simulink model "BG"  (R2014a)
settings: Solver=ode3  StartTime=0.0  StopTime=1  FixedStep=dt  MaxStep=dt  RelTol=1e-3
values from neighbouring files (symbols this model uses):
  a1 = .4    (= 0.4)    [parameters.m]
  a2 = .35    (= 0.35)    [parameters.m]
  a3 = .25    (= 0.25)    [parameters.m]
  aTc = 0.05    [parameters.m]
  dt = 1e-3    (= 0.001)    [parameters.m]
  g = 1    [parameters.m]
  K = 1    [parameters.m]
  mTc = 0.01    [parameters.m]
  OP1_0 = [ax1_0 ay1_0 0]    [parameters.m]
  OP2_0 = OP1_0 + P1P2_0    [parameters.m]
  OP3_0 = OP2_0 + P2P3_0    [parameters.m]
  OT = [xf yf 0]    [animation.m]    (also in parameters.m = [0.5 0.5 0])
  OT_cercle = [0.6 0.55 0]    [parameters.m]
  p1 = w2 + w3    (= 3)    [parameters.m]
  P1P2_0 = [ax2_0 ay2_0 0]    [parameters.m]
  p2 = w1 + w3    (= 4)    [parameters.m]
  P2P3_0 = [ax3_0 ay3_0 0]    [parameters.m]
  p3 = w2 + w1    (= 5)    [parameters.m]
  tau = 0.001    [parameters.m]
  theta1_0 = zero_vector    [parameters.m]
  theta2_0 = zero_vector    [parameters.m]
  theta3_0 = zero_vector    [parameters.m]
  Vmax = 30    [parameters.m]
  w1 = 3    [parameters.m]
  w2 = 2    [parameters.m]
  w3 = 1    [parameters.m]
  zero_vector = [0 0 0]    [parameters.m]
libraries: vrlib x9, simulink x1
(part 3 of 4)

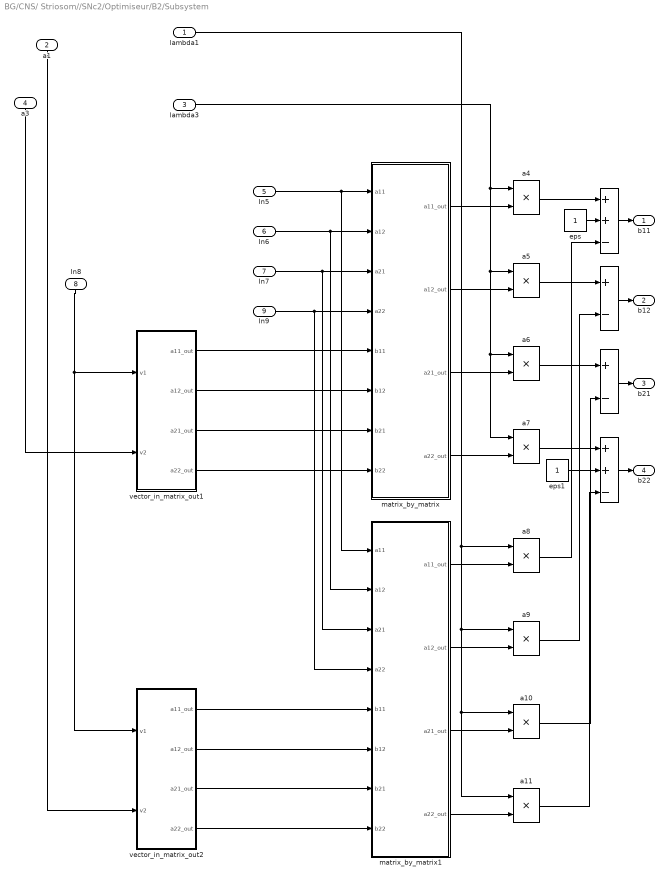
== system BG/CNS/ Striosom//SNc2/Optimiseur/B2/Subsystem ==
  lambda1 : Inport
  a1 : Inport  Port=2
  lambda3 : Inport  Port=3
  a3 : Inport  Port=4
  In5 : Inport  Port=5
  In6 : Inport  Port=6
  In7 : Inport  Port=7
  In8 : Inport  Port=8
  In9 : Inport  Port=9
  "                                                                                                    " : Sum  Inputs=++-
  "                                                                                                      " : Sum  Inputs=++-
  "                                                                                                       " : Sum  Inputs=+-
  "                                                                                                           " : Sum  Inputs=+-
  a{4..11} (8 alike) : Product
  eps : Constant
  eps1 : Constant
  matrix_by_matrix : Subsystem
  matrix_by_matrix1 : Subsystem
  vector_in_matrix_out1 : Subsystem
  vector_in_matrix_out2 : Subsystem
  b11 : Outport
  b12 : Outport  Port=2
  b21 : Outport  Port=3
  b22 : Outport  Port=4
  wires:
  In5/1 -> matrix_by_matrix1/1(a11), matrix_by_matrix/1(a11)
  In6/1 -> matrix_by_matrix1/2(a12), matrix_by_matrix/2(a12)
  In7/1 -> matrix_by_matrix1/3(a21), matrix_by_matrix/3(a21)
  In9/1 -> matrix_by_matrix1/4(a22), matrix_by_matrix/4(a22)
  vector_in_matrix_out1/4(a22_out) -> matrix_by_matrix/8(b22)
  vector_in_matrix_out1/3(a21_out) -> matrix_by_matrix/7(b21)
  vector_in_matrix_out1/1(a11_out) -> matrix_by_matrix/5(b11)
  vector_in_matrix_out1/2(a12_out) -> matrix_by_matrix/6(b12)
  matrix_by_matrix/1(a11_out) -> a4/2
  lambda3/1 -> a7/1, a6/1, a5/1, a4/1
  matrix_by_matrix/2(a12_out) -> a5/2
  matrix_by_matrix/3(a21_out) -> a6/2
  matrix_by_matrix/4(a22_out) -> a7/2
  vector_in_matrix_out2/2(a12_out) -> matrix_by_matrix1/6(b12)
  vector_in_matrix_out2/3(a21_out) -> matrix_by_matrix1/7(b21)
  vector_in_matrix_out2/1(a11_out) -> matrix_by_matrix1/5(b11)
  vector_in_matrix_out2/4(a22_out) -> matrix_by_matrix1/8(b22)
  matrix_by_matrix1/1(a11_out) -> a8/2
  matrix_by_matrix1/2(a12_out) -> a9/2
  matrix_by_matrix1/3(a21_out) -> a10/2
  matrix_by_matrix1/4(a22_out) -> a11/2
  lambda1/1 -> a11/1, a10/1, a9/1, a8/1
  a4/1 -> "                                                                                                    "/1
  a8/1 -> "                                                                                                    "/3
  eps/1 -> "                                                                                                    "/2
  a5/1 -> "                                                                                                       "/1
  a9/1 -> "                                                                                                       "/2
  a6/1 -> "                                                                                                           "/1
  a10/1 -> "                                                                                                           "/2
  a7/1 -> "                                                                                                      "/1
  eps1/1 -> "                                                                                                      "/2
  a11/1 -> "                                                                                                      "/3
  a1/1 -> vector_in_matrix_out2/2(v2)
  "                                                                                                       "/1 -> b12/1
  "                                                                                                           "/1 -> b21/1
  a3/1 -> vector_in_matrix_out1/2(v2)
  "                                                                                                      "/1 -> b22/1
  "                                                                                                    "/1 -> b11/1
  In8/1 -> vector_in_matrix_out2/1(v1), vector_in_matrix_out1/1(v1)

== system BG/CNS/ Striosom//SNc2/Optimiseur/B2/inverse_matrix ==
  a11 : Inport
  a12 : Inport  Port=2
  a21 : Inport  Port=3
  a22 : Inport  Port=4
  "                                                                                                    " : Sum  Inputs=+-+
  Divide{1..4} (4 alike) : Product  Inputs=*/
  Gain : Gain  Gain=-1
  Gain1 : Gain  Gain=-1
  a1 : Product
  a2 : Product
  eps : Constant  Value=1e-4
  a11_out : Outport
  a12_out : Outport  Port=2
  a21_out : Outport  Port=3
  a22_out : Outport  Port=4
  wires:
  a11/1 -> Divide2/1, a1/1
  a22/1 -> Divide1/1, a1/2
  a12/1 -> a2/1, Gain1/1
  a21/1 -> Gain/1, a2/2
  a1/1 -> "                                                                                                    "/1
  a2/1 -> "                                                                                                    "/2
  "                                                                                                    "/1 -> Divide1/2, Divide2/2, Divide3/2, Divide4/2
  Divide1/1 -> a11_out/1
  Divide2/1 -> a22_out/1
  Divide3/1 -> a12_out/1
  Divide4/1 -> a21_out/1
  Gain/1 -> Divide4/1
  Gain1/1 -> Divide3/1
  eps/1 -> "                                                                                                    "/3

== system BG/CNS/ Striosom//SNc2/Optimiseur/B2/vector_in_matrix_out ==
  v1 : Inport
  v2 : Inport  Port=2
  Demux : Demux  Outputs=3
  Demux1 : Demux  Outputs=3
  a{11..12,21..22} (4 alike) : Product
  a11_out : Outport
  a12_out : Outport  Port=2
  a21_out : Outport  Port=3
  a22_out : Outport  Port=4
  wires:
  v1/1 -> Demux/1
  v2/1 -> Demux1/1
  a11/1 -> a11_out/1
  Demux/1 -> a12/1, a11/1
  a12/1 -> a12_out/1
  a21/1 -> a21_out/1
  Demux/2 -> a22/1, a21/1
  a22/1 -> a22_out/1
  Demux1/1 -> a11/2, a21/2
  Demux1/2 -> a22/2, a12/2

== system BG/CNS/ Striosom//SNc2/Optimiseur/lambda/alpha ==
  d : Inport
  c1 : Inport  Port=2
  c2 : Inport  Port=3
  c3 : Inport  Port=4
  "                                                                                                    " : Sum
  Divide1 : Product  Inputs=*/
  Divide2 : Product  Inputs=*/
  Divide3 : Product  Inputs=*/
  Gain : Gain  Gain=w2*w3
  Gain1 : Gain  Gain=w1*w3
  Gain2 : Gain  Gain=w2*w1
  eps : Constant  Value=1e-2
  alpha1 : Outport
  alpha2 : Outport  Port=2
  alpha3 : Outport  Port=3
  wires:
  c1/1 -> Divide1/1
  d/1 -> "                                                                                                    "/1
  eps/1 -> "                                                                                                    "/2
  Divide1/1 -> Gain/1
  "                                                                                                    "/1 -> Divide3/2, Divide2/2, Divide1/2
  c2/1 -> Divide2/1
  Divide2/1 -> Gain1/1
  Divide3/1 -> Gain2/1
  c3/1 -> Divide3/1
  Gain/1 -> alpha1/1
  Gain1/1 -> alpha2/1
  Gain2/1 -> alpha3/1

== system BG/CNS/ Striosom//SNc2/Optimiseur/lambda/d=V^T(VV^T)^-1V ==
  In1 : Inport
  Dot Product : DotProduct  InputSameDT=on  OutDataTypeStr=Inherit: Inherit via internal rule
  inverse_matrix : Subsystem
  matrix_vector_multiplication : Subsystem
  vector_in_matrix_out : Subsystem
  d : Outport
  wires:
  vector_in_matrix_out/4(a22_out) -> inverse_matrix/4(a22)
  vector_in_matrix_out/2(a12_out) -> inverse_matrix/2(a12)
  vector_in_matrix_out/1(a11_out) -> inverse_matrix/1(a11)
  matrix_vector_multiplication/1(vec_out) -> Dot Product/2
  vector_in_matrix_out/3(a21_out) -> inverse_matrix/3(a21)
  inverse_matrix/2(a12_out) -> matrix_vector_multiplication/2(a12)
  In1/1 -> Dot Product/1, matrix_vector_multiplication/5(v1), vector_in_matrix_out/2(v2), vector_in_matrix_out/1(v1)
  inverse_matrix/3(a21_out) -> matrix_vector_multiplication/3(a21)
  inverse_matrix/1(a11_out) -> matrix_vector_multiplication/1(a11)
  inverse_matrix/4(a22_out) -> matrix_vector_multiplication/4(a22)
  Dot Product/1 -> d/1

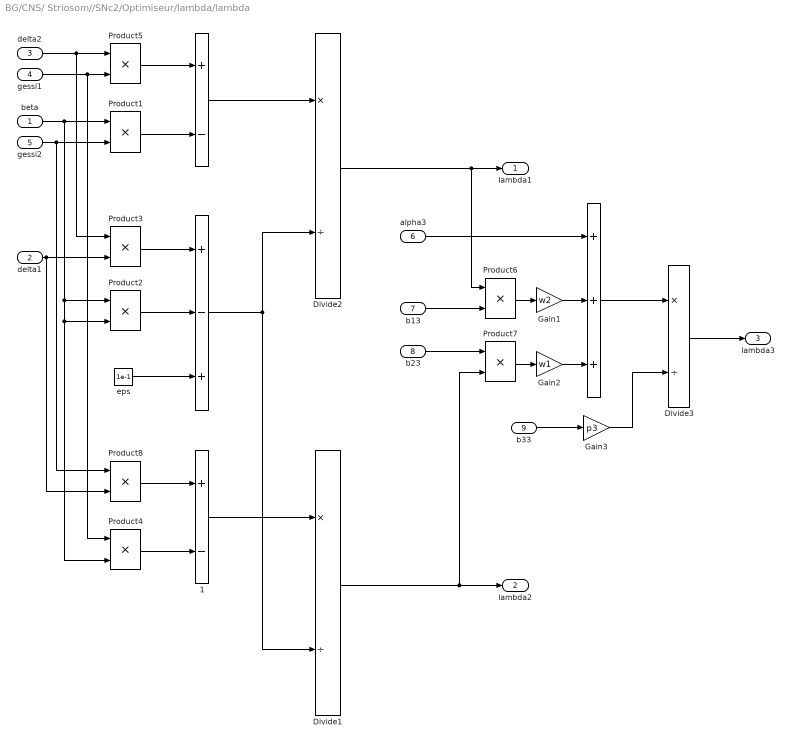
== system BG/CNS/ Striosom//SNc2/Optimiseur/lambda/lambda ==
  beta : Inport
  delta1 : Inport  Port=2
  delta2 : Inport  Port=3
  gessi1 : Inport  Port=4
  gessi2 : Inport  Port=5
  alpha3 : Inport  Port=6
  b13 : Inport  Port=7
  b23 : Inport  Port=8
  b33 : Inport  Port=9
  "                                                                                                        " : Sum  Inputs=+-
  "                                                                                                           " : Sum  Inputs=+-+
  "                                                                                                                 " : Sum  Inputs=+++
  "                                                                                                        1" : Sum  Inputs=+-
  Divide1 : Product  Inputs=*/
  Divide2 : Product  Inputs=*/
  Divide3 : Product  Inputs=*/
  Gain1 : Gain  Gain=w2
  Gain2 : Gain  Gain=w1
  Gain3 : Gain  Gain=p3
  Product{1..8} (8 alike) : Product
  eps : Constant  Value=1e-1
  lambda1 : Outport
  lambda2 : Outport  Port=2
  lambda3 : Outport  Port=3
  wires:
  delta2/1 -> Product3/1, Product5/1
  Product5/1 -> "                                                                                                        "/1
  Product1/1 -> "                                                                                                        "/2
  Product3/1 -> "                                                                                                           "/1
  Product2/1 -> "                                                                                                           "/2
  eps/1 -> "                                                                                                           "/3
  "                                                                                                        "/1 -> Divide2/1
  "                                                                                                           "/1 -> Divide2/2, Divide1/2
  Divide2/1 -> Product6/1, lambda1/1
  gessi2/1 -> Product8/1, Product1/2
  delta1/1 -> Product8/2, Product3/2
  gessi1/1 -> Product4/1, Product5/2
  beta/1 -> Product2/2, Product4/2, Product2/1, Product1/1
  Product8/1 -> "                                                                                                        1"/1
  Product4/1 -> "                                                                                                        1"/2
  "                                                                                                        1"/1 -> Divide1/1
  Divide1/1 -> Product7/2, lambda2/1
  b13/1 -> Product6/2
  b23/1 -> Product7/1
  Product7/1 -> Gain2/1
  Product6/1 -> Gain1/1
  alpha3/1 -> "                                                                                                                 "/1
  "                                                                                                                 "/1 -> Divide3/1
  b33/1 -> Gain3/1
  Gain3/1 -> Divide3/2
  Divide3/1 -> lambda3/1
  Gain1/1 -> "                                                                                                                 "/2
  Gain2/1 -> "                                                                                                                 "/3

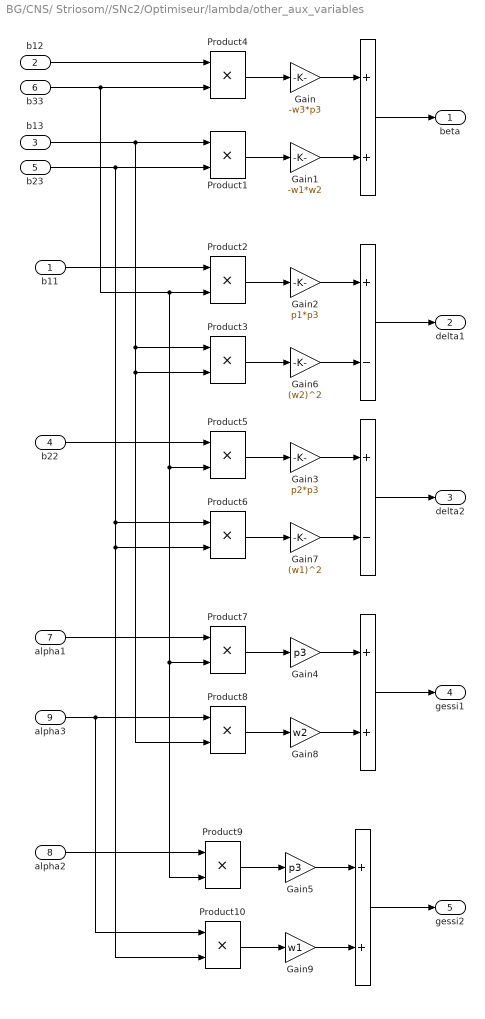
== system BG/CNS/ Striosom//SNc2/Optimiseur/lambda/other_aux_variables ==
  b11 : Inport
  b12 : Inport  Port=2
  b13 : Inport  Port=3
  b22 : Inport  Port=4
  b23 : Inport  Port=5
  b33 : Inport  Port=6
  alpha1 : Inport  Port=7
  alpha2 : Inport  Port=8
  alpha3 : Inport  Port=9
  "                                                                                                    " : Sum
  "                                                                                                     " : Sum  Inputs=+-
  "                                                                                                        " : Sum  Inputs=+-
  "                                                                                                                          " : Sum
  "                                                                                                                               " : Sum
  Gain : Gain  Gain=-w3*p3
  Gain1 : Gain  Gain=-w1*w2
  Gain2 : Gain  Gain=p1*p3
  Gain3 : Gain  Gain=p2*p3
  Gain4 : Gain  Gain=p3
  Gain5 : Gain  Gain=p3
  Gain6 : Gain  Gain=(w2)^2
  Gain7 : Gain  Gain=(w1)^2
  Gain8 : Gain  Gain=w2
  Gain9 : Gain  Gain=w1
  Product{1..10} (10 alike) : Product
  beta : Outport
  delta1 : Outport  Port=2
  delta2 : Outport  Port=3
  gessi1 : Outport  Port=4
  gessi2 : Outport  Port=5
  wires:
  b12/1 -> Product4/1
  Product4/1 -> Gain/1
  Product1/1 -> Gain1/1
  Gain/1 -> "                                                                                                    "/1
  Gain1/1 -> "                                                                                                    "/2
  "                                                                                                    "/1 -> beta/1
  Product2/1 -> Gain2/1
  b11/1 -> Product2/1
  Gain2/1 -> "                                                                                                     "/1
  Product3/1 -> Gain6/1
  "                                                                                                     "/1 -> delta1/1
  b23/1 -> Product6/1, Product10/2, Product6/2, Product1/2
  Product5/1 -> Gain3/1
  b22/1 -> Product5/1
  Gain3/1 -> "                                                                                                        "/1
  Product6/1 -> Gain7/1
  "                                                                                                        "/1 -> delta2/1
  b33/1 -> Product9/2, Product7/2, Product5/2, Product2/2, Product4/2
  alpha3/1 -> Product10/1, Product8/1
  b13/1 -> Product8/2, Product3/2, Product3/1, Product1/1
  Product7/1 -> Gain4/1
  alpha1/1 -> Product7/1
  Gain4/1 -> "                                                                                                                          "/1
  Product8/1 -> Gain8/1
  "                                                                                                                          "/1 -> gessi1/1
  Product9/1 -> Gain5/1
  Gain5/1 -> "                                                                                                                               "/1
  Product10/1 -> Gain9/1
  "                                                                                                                               "/1 -> gessi2/1
  alpha2/1 -> Product9/1
  Gain6/1 -> "                                                                                                     "/2
  Gain7/1 -> "                                                                                                        "/2
  Gain8/1 -> "                                                                                                                          "/2
  Gain9/1 -> "                                                                                                                               "/2

== system BG/CNS/ Striosom//SNc2/Optimiseur/lambda/producing_dot_productions ==
  v : Inport
  a1 : Inport  Port=2
  a2 : Inport  Port=3
  a3 : Inport  Port=4
  Dot Product{,1..8} (9 alike) : DotProduct  InputSameDT=on  OutDataTypeStr=Inherit: Inherit via internal rule
  c1 : Outport
  c2 : Outport  Port=2
  c3 : Outport  Port=3
  b11 : Outport  Port=4
  b12 : Outport  Port=5
  b13 : Outport  Port=6
  b22 : Outport  Port=7
  b23 : Outport  Port=8
  b33 : Outport  Port=9
  wires:
  Dot Product/1 -> c1/1
  v/1 -> Dot Product2/1, Dot Product1/1, Dot Product/1
  a1/1 -> Dot Product4/1, Dot Product5/1, Dot Product3/2, Dot Product3/1, Dot Product/2
  Dot Product1/1 -> c2/1
  a2/1 -> Dot Product7/1, Dot Product6/2, Dot Product6/1, Dot Product4/2, Dot Product1/2
  Dot Product2/1 -> c3/1
  a3/1 -> Dot Product5/2, Dot Product7/2, Dot Product8/1, Dot Product8/2, Dot Product2/2
  Dot Product3/1 -> b11/1
  Dot Product4/1 -> b12/1
  Dot Product5/1 -> b13/1
  Dot Product6/1 -> b22/1
  Dot Product7/1 -> b23/1
  Dot Product8/1 -> b33/1

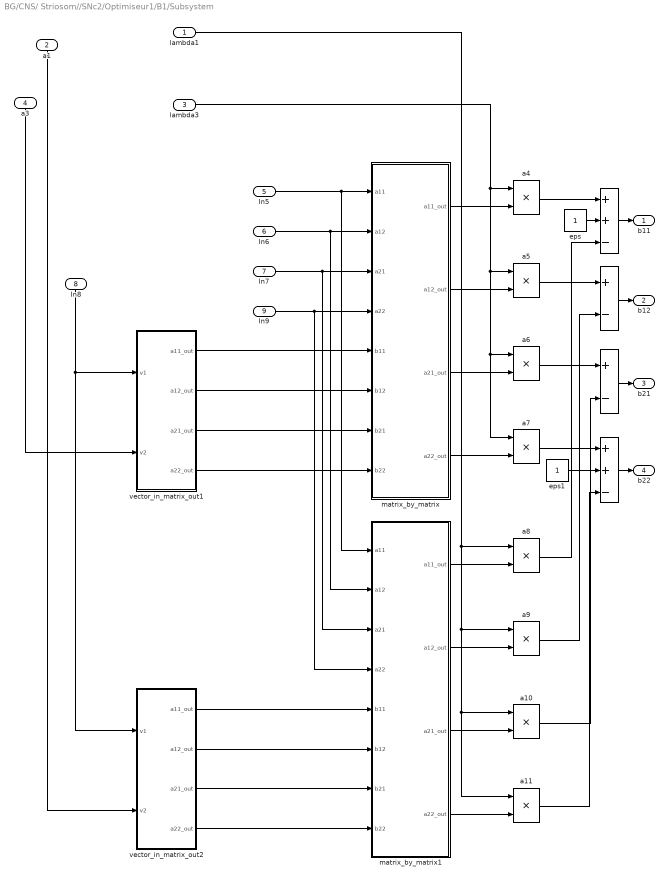
== system BG/CNS/ Striosom//SNc2/Optimiseur1/B1/Subsystem ==
  lambda1 : Inport
  a1 : Inport  Port=2
  lambda3 : Inport  Port=3
  a3 : Inport  Port=4
  In5 : Inport  Port=5
  In6 : Inport  Port=6
  In7 : Inport  Port=7
  In8 : Inport  Port=8
  In9 : Inport  Port=9
  "                                                                                                    " : Sum  Inputs=++-
  "                                                                                                      " : Sum  Inputs=++-
  "                                                                                                       " : Sum  Inputs=+-
  "                                                                                                           " : Sum  Inputs=+-
  a{4..11} (8 alike) : Product
  eps : Constant
  eps1 : Constant
  matrix_by_matrix : Subsystem
  matrix_by_matrix1 : Subsystem
  vector_in_matrix_out1 : Subsystem
  vector_in_matrix_out2 : Subsystem
  b11 : Outport
  b12 : Outport  Port=2
  b21 : Outport  Port=3
  b22 : Outport  Port=4
  wires:
  In5/1 -> matrix_by_matrix1/1(a11), matrix_by_matrix/1(a11)
  In6/1 -> matrix_by_matrix1/2(a12), matrix_by_matrix/2(a12)
  In7/1 -> matrix_by_matrix1/3(a21), matrix_by_matrix/3(a21)
  In9/1 -> matrix_by_matrix1/4(a22), matrix_by_matrix/4(a22)
  vector_in_matrix_out1/4(a22_out) -> matrix_by_matrix/8(b22)
  vector_in_matrix_out1/3(a21_out) -> matrix_by_matrix/7(b21)
  vector_in_matrix_out1/1(a11_out) -> matrix_by_matrix/5(b11)
  vector_in_matrix_out1/2(a12_out) -> matrix_by_matrix/6(b12)
  matrix_by_matrix/1(a11_out) -> a4/2
  lambda3/1 -> a7/1, a6/1, a5/1, a4/1
  matrix_by_matrix/2(a12_out) -> a5/2
  matrix_by_matrix/3(a21_out) -> a6/2
  matrix_by_matrix/4(a22_out) -> a7/2
  vector_in_matrix_out2/2(a12_out) -> matrix_by_matrix1/6(b12)
  vector_in_matrix_out2/3(a21_out) -> matrix_by_matrix1/7(b21)
  vector_in_matrix_out2/1(a11_out) -> matrix_by_matrix1/5(b11)
  vector_in_matrix_out2/4(a22_out) -> matrix_by_matrix1/8(b22)
  matrix_by_matrix1/1(a11_out) -> a8/2
  matrix_by_matrix1/2(a12_out) -> a9/2
  matrix_by_matrix1/3(a21_out) -> a10/2
  matrix_by_matrix1/4(a22_out) -> a11/2
  lambda1/1 -> a11/1, a10/1, a9/1, a8/1
  a4/1 -> "                                                                                                    "/1
  a8/1 -> "                                                                                                    "/3
  eps/1 -> "                                                                                                    "/2
  a5/1 -> "                                                                                                       "/1
  a9/1 -> "                                                                                                       "/2
  a6/1 -> "                                                                                                           "/1
  a10/1 -> "                                                                                                           "/2
  a7/1 -> "                                                                                                      "/1
  eps1/1 -> "                                                                                                      "/2
  a11/1 -> "                                                                                                      "/3
  a1/1 -> vector_in_matrix_out2/2(v2)
  "                                                                                                       "/1 -> b12/1
  "                                                                                                           "/1 -> b21/1
  a3/1 -> vector_in_matrix_out1/2(v2)
  "                                                                                                      "/1 -> b22/1
  "                                                                                                    "/1 -> b11/1
  In8/1 -> vector_in_matrix_out2/1(v1), vector_in_matrix_out1/1(v1)

== system BG/CNS/ Striosom//SNc2/Optimiseur1/B1/inverse_matrix ==
  a11 : Inport
  a12 : Inport  Port=2
  a21 : Inport  Port=3
  a22 : Inport  Port=4
  "                                                                                                    " : Sum  Inputs=+-+
  Divide{1..4} (4 alike) : Product  Inputs=*/
  Gain : Gain  Gain=-1
  Gain1 : Gain  Gain=-1
  a1 : Product
  a2 : Product
  eps : Constant  Value=1e-3
  a11_out : Outport
  a12_out : Outport  Port=2
  a21_out : Outport  Port=3
  a22_out : Outport  Port=4
  wires:
  a11/1 -> Divide2/1, a1/1
  a22/1 -> Divide1/1, a1/2
  a12/1 -> a2/1, Gain1/1
  a21/1 -> Gain/1, a2/2
  a1/1 -> "                                                                                                    "/1
  a2/1 -> "                                                                                                    "/2
  "                                                                                                    "/1 -> Divide1/2, Divide2/2, Divide3/2, Divide4/2
  Divide1/1 -> a11_out/1
  Divide2/1 -> a22_out/1
  Divide3/1 -> a12_out/1
  Divide4/1 -> a21_out/1
  Gain/1 -> Divide4/1
  Gain1/1 -> Divide3/1
  eps/1 -> "                                                                                                    "/3

== system BG/CNS/ Striosom//SNc2/Optimiseur1/B1/vector_in_matrix_out ==
  v1 : Inport
  v2 : Inport  Port=2
  Demux : Demux  Outputs=3
  Demux1 : Demux  Outputs=3
  a{11..12,21..22} (4 alike) : Product
  a11_out : Outport
  a12_out : Outport  Port=2
  a21_out : Outport  Port=3
  a22_out : Outport  Port=4
  wires:
  v1/1 -> Demux/1
  v2/1 -> Demux1/1
  a11/1 -> a11_out/1
  Demux/1 -> a12/1, a11/1
  a12/1 -> a12_out/1
  a21/1 -> a21_out/1
  Demux/2 -> a22/1, a21/1
  a22/1 -> a22_out/1
  Demux1/1 -> a11/2, a21/2
  Demux1/2 -> a22/2, a12/2

== system BG/CNS/ Striosom//SNc2/Optimiseur1/B2/Subsystem ==
  lambda1 : Inport
  a1 : Inport  Port=2
  lambda3 : Inport  Port=3
  a3 : Inport  Port=4
  In5 : Inport  Port=5
  In6 : Inport  Port=6
  In7 : Inport  Port=7
  In8 : Inport  Port=8
  In9 : Inport  Port=9
  "                                                                                                    " : Sum  Inputs=++-
  "                                                                                                      " : Sum  Inputs=++-
  "                                                                                                       " : Sum  Inputs=+-
  "                                                                                                           " : Sum  Inputs=+-
  a{4..11} (8 alike) : Product
  eps : Constant
  eps1 : Constant
  matrix_by_matrix : Subsystem
  matrix_by_matrix1 : Subsystem
  vector_in_matrix_out1 : Subsystem
  vector_in_matrix_out2 : Subsystem
  b11 : Outport
  b12 : Outport  Port=2
  b21 : Outport  Port=3
  b22 : Outport  Port=4
  wires:
  In5/1 -> matrix_by_matrix1/1(a11), matrix_by_matrix/1(a11)
  In6/1 -> matrix_by_matrix1/2(a12), matrix_by_matrix/2(a12)
  In7/1 -> matrix_by_matrix1/3(a21), matrix_by_matrix/3(a21)
  In9/1 -> matrix_by_matrix1/4(a22), matrix_by_matrix/4(a22)
  vector_in_matrix_out1/4(a22_out) -> matrix_by_matrix/8(b22)
  vector_in_matrix_out1/3(a21_out) -> matrix_by_matrix/7(b21)
  vector_in_matrix_out1/1(a11_out) -> matrix_by_matrix/5(b11)
  vector_in_matrix_out1/2(a12_out) -> matrix_by_matrix/6(b12)
  matrix_by_matrix/1(a11_out) -> a4/2
  lambda3/1 -> a7/1, a6/1, a5/1, a4/1
  matrix_by_matrix/2(a12_out) -> a5/2
  matrix_by_matrix/3(a21_out) -> a6/2
  matrix_by_matrix/4(a22_out) -> a7/2
  vector_in_matrix_out2/2(a12_out) -> matrix_by_matrix1/6(b12)
  vector_in_matrix_out2/3(a21_out) -> matrix_by_matrix1/7(b21)
  vector_in_matrix_out2/1(a11_out) -> matrix_by_matrix1/5(b11)
  vector_in_matrix_out2/4(a22_out) -> matrix_by_matrix1/8(b22)
  matrix_by_matrix1/1(a11_out) -> a8/2
  matrix_by_matrix1/2(a12_out) -> a9/2
  matrix_by_matrix1/3(a21_out) -> a10/2
  matrix_by_matrix1/4(a22_out) -> a11/2
  lambda1/1 -> a11/1, a10/1, a9/1, a8/1
  a4/1 -> "                                                                                                    "/1
  a8/1 -> "                                                                                                    "/3
  eps/1 -> "                                                                                                    "/2
  a5/1 -> "                                                                                                       "/1
  a9/1 -> "                                                                                                       "/2
  a6/1 -> "                                                                                                           "/1
  a10/1 -> "                                                                                                           "/2
  a7/1 -> "                                                                                                      "/1
  eps1/1 -> "                                                                                                      "/2
  a11/1 -> "                                                                                                      "/3
  a1/1 -> vector_in_matrix_out2/2(v2)
  "                                                                                                       "/1 -> b12/1
  "                                                                                                           "/1 -> b21/1
  a3/1 -> vector_in_matrix_out1/2(v2)
  "                                                                                                      "/1 -> b22/1
  "                                                                                                    "/1 -> b11/1
  In8/1 -> vector_in_matrix_out2/1(v1), vector_in_matrix_out1/1(v1)

== system BG/CNS/ Striosom//SNc2/Optimiseur1/B2/inverse_matrix ==
  a11 : Inport
  a12 : Inport  Port=2
  a21 : Inport  Port=3
  a22 : Inport  Port=4
  "                                                                                                    " : Sum  Inputs=+-+
  Divide{1..4} (4 alike) : Product  Inputs=*/
  Gain : Gain  Gain=-1
  Gain1 : Gain  Gain=-1
  a1 : Product
  a2 : Product
  eps : Constant  Value=1e-3
  a11_out : Outport
  a12_out : Outport  Port=2
  a21_out : Outport  Port=3
  a22_out : Outport  Port=4
  wires:
  a11/1 -> Divide2/1, a1/1
  a22/1 -> Divide1/1, a1/2
  a12/1 -> a2/1, Gain1/1
  a21/1 -> Gain/1, a2/2
  a1/1 -> "                                                                                                    "/1
  a2/1 -> "                                                                                                    "/2
  "                                                                                                    "/1 -> Divide1/2, Divide2/2, Divide3/2, Divide4/2
  Divide1/1 -> a11_out/1
  Divide2/1 -> a22_out/1
  Divide3/1 -> a12_out/1
  Divide4/1 -> a21_out/1
  Gain/1 -> Divide4/1
  Gain1/1 -> Divide3/1
  eps/1 -> "                                                                                                    "/3

== system BG/CNS/ Striosom//SNc2/Optimiseur1/B2/vector_in_matrix_out ==
  v1 : Inport
  v2 : Inport  Port=2
  Demux : Demux  Outputs=3
  Demux1 : Demux  Outputs=3
  a{11..12,21..22} (4 alike) : Product
  a11_out : Outport
  a12_out : Outport  Port=2
  a21_out : Outport  Port=3
  a22_out : Outport  Port=4
  wires:
  v1/1 -> Demux/1
  v2/1 -> Demux1/1
  a11/1 -> a11_out/1
  Demux/1 -> a12/1, a11/1
  a12/1 -> a12_out/1
  a21/1 -> a21_out/1
  Demux/2 -> a22/1, a21/1
  a22/1 -> a22_out/1
  Demux1/1 -> a11/2, a21/2
  Demux1/2 -> a22/2, a12/2

== system BG/CNS/ Striosom//SNc2/Optimiseur1/lambda/alpha ==
  d : Inport
  c1 : Inport  Port=2
  c2 : Inport  Port=3
  c3 : Inport  Port=4
  "                                                                                                    " : Sum
  Divide1 : Product  Inputs=*/
  Divide2 : Product  Inputs=*/
  Divide3 : Product  Inputs=*/
  eps : Constant  Value=1e-4
  alpha1 : Outport
  alpha2 : Outport  Port=2
  alpha3 : Outport  Port=3
  wires:
  c1/1 -> Divide1/1
  d/1 -> "                                                                                                    "/1
  eps/1 -> "                                                                                                    "/2
  Divide1/1 -> alpha1/1
  "                                                                                                    "/1 -> Divide3/2, Divide2/2, Divide1/2
  c2/1 -> Divide2/1
  Divide2/1 -> alpha2/1
  Divide3/1 -> alpha3/1
  c3/1 -> Divide3/1

== system BG/CNS/ Striosom//SNc2/Optimiseur1/lambda/d=V^T(VV^T)^-1V ==
  In1 : Inport
  Dot Product : DotProduct  InputSameDT=on  OutDataTypeStr=Inherit: Inherit via internal rule
  inverse_matrix : Subsystem
  matrix_vector_multiplication : Subsystem
  vector_in_matrix_out : Subsystem
  d : Outport
  wires:
  vector_in_matrix_out/4(a22_out) -> inverse_matrix/4(a22)
  vector_in_matrix_out/2(a12_out) -> inverse_matrix/2(a12)
  vector_in_matrix_out/1(a11_out) -> inverse_matrix/1(a11)
  matrix_vector_multiplication/1(vec_out) -> Dot Product/2
  vector_in_matrix_out/3(a21_out) -> inverse_matrix/3(a21)
  inverse_matrix/2(a12_out) -> matrix_vector_multiplication/2(a12)
  In1/1 -> Dot Product/1, matrix_vector_multiplication/5(v1), vector_in_matrix_out/2(v2), vector_in_matrix_out/1(v1)
  inverse_matrix/3(a21_out) -> matrix_vector_multiplication/3(a21)
  inverse_matrix/1(a11_out) -> matrix_vector_multiplication/1(a11)
  inverse_matrix/4(a22_out) -> matrix_vector_multiplication/4(a22)
  Dot Product/1 -> d/1

== system BG/CNS/ Striosom//SNc2/Optimiseur1/lambda/lambda ==
  beta : Inport
  delta1 : Inport  Port=2
  delta2 : Inport  Port=3
  gessi1 : Inport  Port=4
  gessi2 : Inport  Port=5
  alpha3 : Inport  Port=6
  b13 : Inport  Port=7
  b23 : Inport  Port=8
  b33 : Inport  Port=9
  "                                                                                                        " : Sum  Inputs=+-
  "                                                                                                           " : Sum  Inputs=+-+
  "                                                                                                                 " : Sum  Inputs=+++
  "                                                                                                        1" : Sum  Inputs=+-
  Divide1 : Product  Inputs=*/
  Divide2 : Product  Inputs=*/
  Divide3 : Product  Inputs=*/
  Gain3 : Gain  Gain=2
  Product{1..8} (8 alike) : Product
  eps : Constant  Value=1e-4
  lambda1 : Outport
  lambda2 : Outport  Port=2
  lambda3 : Outport  Port=3
  wires:
  delta2/1 -> Product3/1, Product5/1
  Product5/1 -> "                                                                                                        "/1
  Product1/1 -> "                                                                                                        "/2
  Product3/1 -> "                                                                                                           "/1
  Product2/1 -> "                                                                                                           "/2
  eps/1 -> "                                                                                                           "/3
  "                                                                                                        "/1 -> Divide2/1
  "                                                                                                           "/1 -> Divide2/2, Divide1/2
  Divide2/1 -> Product6/1, lambda1/1
  gessi2/1 -> Product8/1, Product1/2
  delta1/1 -> Product8/2, Product3/2
  gessi1/1 -> Product4/1, Product5/2
  beta/1 -> Product2/2, Product4/2, Product2/1, Product1/1
  Product8/1 -> "                                                                                                        1"/1
  Product4/1 -> "                                                                                                        1"/2
  "                                                                                                        1"/1 -> Divide1/1
  Divide1/1 -> Product7/2, lambda2/1
  b13/1 -> Product6/2
  b23/1 -> Product7/1
  Product7/1 -> "                                                                                                                 "/3
  Product6/1 -> "                                                                                                                 "/2
  alpha3/1 -> "                                                                                                                 "/1
  "                                                                                                                 "/1 -> Divide3/1
  b33/1 -> Gain3/1
  Gain3/1 -> Divide3/2
  Divide3/1 -> lambda3/1

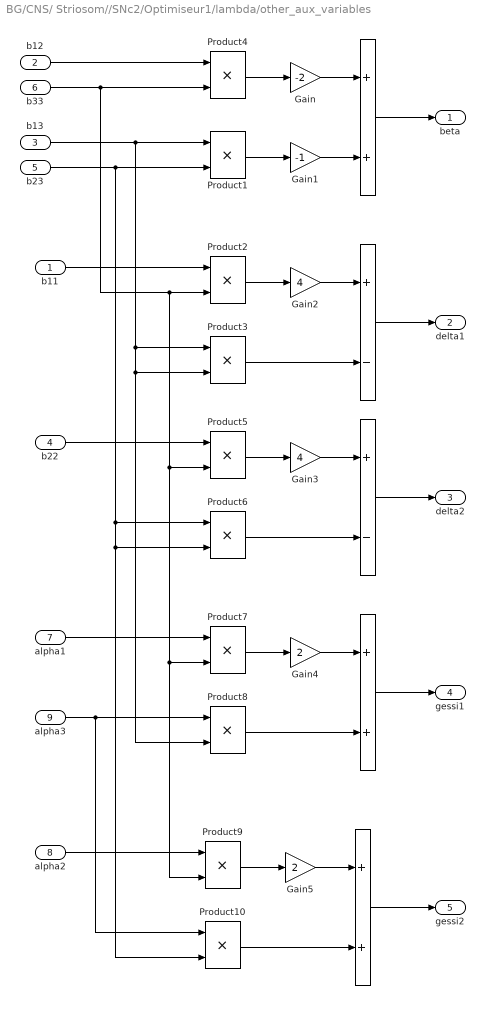
== system BG/CNS/ Striosom//SNc2/Optimiseur1/lambda/other_aux_variables ==
  b11 : Inport
  b12 : Inport  Port=2
  b13 : Inport  Port=3
  b22 : Inport  Port=4
  b23 : Inport  Port=5
  b33 : Inport  Port=6
  alpha1 : Inport  Port=7
  alpha2 : Inport  Port=8
  alpha3 : Inport  Port=9
  "                                                                                                    " : Sum
  "                                                                                                     " : Sum  Inputs=+-
  "                                                                                                        " : Sum  Inputs=+-
  "                                                                                                                          " : Sum
  "                                                                                                                               " : Sum
  Gain : Gain  Gain=-2
  Gain1 : Gain  Gain=-1
  Gain2 : Gain  Gain=4
  Gain3 : Gain  Gain=4
  Gain4 : Gain  Gain=2
  Gain5 : Gain  Gain=2
  Product{1..10} (10 alike) : Product
  beta : Outport
  delta1 : Outport  Port=2
  delta2 : Outport  Port=3
  gessi1 : Outport  Port=4
  gessi2 : Outport  Port=5
  wires:
  b12/1 -> Product4/1
  Product4/1 -> Gain/1
  Product1/1 -> Gain1/1
  Gain/1 -> "                                                                                                    "/1
  Gain1/1 -> "                                                                                                    "/2
  "                                                                                                    "/1 -> beta/1
  Product2/1 -> Gain2/1
  b11/1 -> Product2/1
  Gain2/1 -> "                                                                                                     "/1
  Product3/1 -> "                                                                                                     "/2
  "                                                                                                     "/1 -> delta1/1
  b23/1 -> Product6/1, Product10/2, Product6/2, Product1/2
  Product5/1 -> Gain3/1
  b22/1 -> Product5/1
  Gain3/1 -> "                                                                                                        "/1
  Product6/1 -> "                                                                                                        "/2
  "                                                                                                        "/1 -> delta2/1
  b33/1 -> Product9/2, Product7/2, Product5/2, Product2/2, Product4/2
  alpha3/1 -> Product10/1, Product8/1
  b13/1 -> Product8/2, Product3/2, Product3/1, Product1/1
  Product7/1 -> Gain4/1
  alpha1/1 -> Product7/1
  Gain4/1 -> "                                                                                                                          "/1
  Product8/1 -> "                                                                                                                          "/2
  "                                                                                                                          "/1 -> gessi1/1
  Product9/1 -> Gain5/1
  Gain5/1 -> "                                                                                                                               "/1
  Product10/1 -> "                                                                                                                               "/2
  "                                                                                                                               "/1 -> gessi2/1
  alpha2/1 -> Product9/1

== system BG/CNS/ Striosom//SNc2/Optimiseur1/lambda/producing_dot_productions ==
  v : Inport
  a1 : Inport  Port=2
  a2 : Inport  Port=3
  a3 : Inport  Port=4
  Dot Product{,1..8} (9 alike) : DotProduct  InputSameDT=on  OutDataTypeStr=Inherit: Inherit via internal rule
  c1 : Outport
  c2 : Outport  Port=2
  c3 : Outport  Port=3
  b11 : Outport  Port=4
  b12 : Outport  Port=5
  b13 : Outport  Port=6
  b22 : Outport  Port=7
  b23 : Outport  Port=8
  b33 : Outport  Port=9
  wires:
  Dot Product/1 -> c1/1
  v/1 -> Dot Product2/1, Dot Product1/1, Dot Product/1
  a1/1 -> Dot Product4/1, Dot Product5/1, Dot Product3/2, Dot Product3/1, Dot Product/2
  Dot Product1/1 -> c2/1
  a2/1 -> Dot Product7/1, Dot Product6/2, Dot Product6/1, Dot Product4/2, Dot Product1/2
  Dot Product2/1 -> c3/1
  a3/1 -> Dot Product5/2, Dot Product7/2, Dot Product8/1, Dot Product8/2, Dot Product2/2
  Dot Product3/1 -> b11/1
  Dot Product4/1 -> b12/1
  Dot Product5/1 -> b13/1
  Dot Product6/1 -> b22/1
  Dot Product7/1 -> b23/1
  Dot Product8/1 -> b33/1

== system BG/CNS/ Striosom//SNc2/Optimiseur/B1/Subsystem/matrix_by_matrix ==
  a11 : Inport
  a12 : Inport  Port=2
  a21 : Inport  Port=3
  a22 : Inport  Port=4
  b11 : Inport  Port=5
  b12 : Inport  Port=6
  b21 : Inport  Port=7
  b22 : Inport  Port=8
  "                                                                                                    " : Sum
  "                                                                                                     " : Sum
  "                                                                                                       " : Sum
  "                                                                                                          " : Sum
  a{1..8} (8 alike) : Product
  a11_out : Outport
  a12_out : Outport  Port=2
  a21_out : Outport  Port=3
  a22_out : Outport  Port=4
  wires:
  a11/1 -> a3/1, a1/1
  b11/1 -> a1/2, a5/2
  a12/1 -> a4/1, a2/1
  a1/1 -> "                                                                                                    "/1
  a2/1 -> "                                                                                                    "/2
  b21/1 -> a6/2, a2/2
  "                                                                                                    "/1 -> a11_out/1
  a3/1 -> "                                                                                                       "/1
  a4/1 -> "                                                                                                       "/2
  "                                                                                                       "/1 -> a12_out/1
  b22/1 -> a8/2, a4/2
  a21/1 -> a5/1, a7/1
  a5/1 -> "                                                                                                     "/1
  a6/1 -> "                                                                                                     "/2
  "                                                                                                     "/1 -> a21_out/1
  a7/1 -> "                                                                                                          "/1
  a8/1 -> "                                                                                                          "/2
  "                                                                                                          "/1 -> a22_out/1
  a22/1 -> a8/1, a6/1
  b12/1 -> a7/2, a3/2

== system BG/CNS/ Striosom//SNc2/Optimiseur/B1/Subsystem/matrix_by_matrix1 ==
  a11 : Inport
  a12 : Inport  Port=2
  a21 : Inport  Port=3
  a22 : Inport  Port=4
  b11 : Inport  Port=5
  b12 : Inport  Port=6
  b21 : Inport  Port=7
  b22 : Inport  Port=8
  "                                                                                                    " : Sum
  "                                                                                                     " : Sum
  "                                                                                                       " : Sum
  "                                                                                                          " : Sum
  a{1..8} (8 alike) : Product
  a11_out : Outport
  a12_out : Outport  Port=2
  a21_out : Outport  Port=3
  a22_out : Outport  Port=4
  wires:
  a11/1 -> a3/1, a1/1
  b11/1 -> a1/2, a5/2
  a12/1 -> a4/1, a2/1
  a1/1 -> "                                                                                                    "/1
  a2/1 -> "                                                                                                    "/2
  b21/1 -> a6/2, a2/2
  "                                                                                                    "/1 -> a11_out/1
  a3/1 -> "                                                                                                       "/1
  a4/1 -> "                                                                                                       "/2
  "                                                                                                       "/1 -> a12_out/1
  b22/1 -> a8/2, a4/2
  a21/1 -> a5/1, a7/1
  a5/1 -> "                                                                                                     "/1
  a6/1 -> "                                                                                                     "/2
  "                                                                                                     "/1 -> a21_out/1
  a7/1 -> "                                                                                                          "/1
  a8/1 -> "                                                                                                          "/2
  "                                                                                                          "/1 -> a22_out/1
  a22/1 -> a8/1, a6/1
  b12/1 -> a7/2, a3/2

== system BG/CNS/ Striosom//SNc2/Optimiseur/B1/Subsystem/vector_in_matrix_out1 ==
  v1 : Inport
  v2 : Inport  Port=2
  Demux : Demux  Outputs=3
  Demux1 : Demux  Outputs=3
  a{11..12,21..22} (4 alike) : Product
  a11_out : Outport
  a12_out : Outport  Port=2
  a21_out : Outport  Port=3
  a22_out : Outport  Port=4
  wires:
  v1/1 -> Demux/1
  v2/1 -> Demux1/1
  a11/1 -> a11_out/1
  Demux/1 -> a12/1, a11/1
  a12/1 -> a12_out/1
  a21/1 -> a21_out/1
  Demux/2 -> a22/1, a21/1
  a22/1 -> a22_out/1
  Demux1/1 -> a11/2, a21/2
  Demux1/2 -> a22/2, a12/2

== system BG/CNS/ Striosom//SNc2/Optimiseur/B1/Subsystem/vector_in_matrix_out2 ==
  v1 : Inport
  v2 : Inport  Port=2
  Demux : Demux  Outputs=3
  Demux1 : Demux  Outputs=3
  a{11..12,21..22} (4 alike) : Product
  a11_out : Outport
  a12_out : Outport  Port=2
  a21_out : Outport  Port=3
  a22_out : Outport  Port=4
  wires:
  v1/1 -> Demux/1
  v2/1 -> Demux1/1
  a11/1 -> a11_out/1
  Demux/1 -> a12/1, a11/1
  a12/1 -> a12_out/1
  a21/1 -> a21_out/1
  Demux/2 -> a22/1, a21/1
  a22/1 -> a22_out/1
  Demux1/1 -> a11/2, a21/2
  Demux1/2 -> a22/2, a12/2

== system BG/CNS/ Striosom//SNc2/Optimiseur/B2/Subsystem/matrix_by_matrix ==
  a11 : Inport
  a12 : Inport  Port=2
  a21 : Inport  Port=3
  a22 : Inport  Port=4
  b11 : Inport  Port=5
  b12 : Inport  Port=6
  b21 : Inport  Port=7
  b22 : Inport  Port=8
  "                                                                                                    " : Sum
  "                                                                                                     " : Sum
  "                                                                                                       " : Sum
  "                                                                                                          " : Sum
  a{1..8} (8 alike) : Product
  a11_out : Outport
  a12_out : Outport  Port=2
  a21_out : Outport  Port=3
  a22_out : Outport  Port=4
  wires:
  a11/1 -> a3/1, a1/1
  b11/1 -> a1/2, a5/2
  a12/1 -> a4/1, a2/1
  a1/1 -> "                                                                                                    "/1
  a2/1 -> "                                                                                                    "/2
  b21/1 -> a6/2, a2/2
  "                                                                                                    "/1 -> a11_out/1
  a3/1 -> "                                                                                                       "/1
  a4/1 -> "                                                                                                       "/2
  "                                                                                                       "/1 -> a12_out/1
  b22/1 -> a8/2, a4/2
  a21/1 -> a5/1, a7/1
  a5/1 -> "                                                                                                     "/1
  a6/1 -> "                                                                                                     "/2
  "                                                                                                     "/1 -> a21_out/1
  a7/1 -> "                                                                                                          "/1
  a8/1 -> "                                                                                                          "/2
  "                                                                                                          "/1 -> a22_out/1
  a22/1 -> a8/1, a6/1
  b12/1 -> a7/2, a3/2
